simulink library "Actuator_AC_Lib"  (R2019b)
settings: Solver=VariableStepAuto  StartTime=0.0  StopTime=10.0  RelTol=1e-3
undefined symbols (not defined in the file): APN_Param
libraries: simulink x3, powerlib x2, electricdrivelib x1
Description:
  | Copyright 2019 The MathWorks, Inc.
settings Model: Creator=smiller  LastModifiedBy=smiller
settings SFSimCC: CustomCodeUndefinedFunction=UseInterfaceOnly

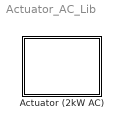
== system Actuator_AC_Lib ==
  Actuator (2kW AC) : Subsystem  VariantControlMode=Label  Variant=on  LabelModeActiveChoice=Phasor  mask{ModelType=Phasor, PQ_Model=Initial}
      mask prompts: ModelType "Model Type"; PQ_Model "PQ Model"
      mask init:
      | set_param(gcb,'LabelModeActiveChoice',get_param(gcb,'ModelType'));
      | set_param([gcb '/Phasor'],'PQ_Model',get_param(gcb,'PQ_Model'));
      settings: AttributesFormatString=%<BlockChoice>
      mask TypeOptions ModelType: Detailed | Phasor
      mask TypeOptions PQ_Model: Initial | Tuned
      mask Display:
      | blk=find_system(gcbh, 'SearchDepth', 1,'FollowLinks','on', 'LookUnderMasks','all', 'Parent', gcb,'VariantObject', get_param(gcb,'activevariant'));
      | eval(get_param(blk, 'MaskDisplay'));

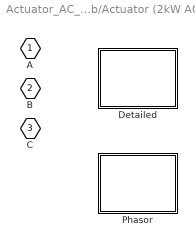
== system Actuator_AC_Lib/Actuator (2kW AC) ==
  Detailed : Subsystem  VariantControl=Detailed
      mask Display: image(imread('ActuatorAC_Detailed_IMAGE.jpg'));
  Phasor : Subsystem  VariantControl=Phasor  mask{PQ_Model=Initial}
      mask prompts: PQ_Model "PQ Model"
      mask init:
      | set_param([gcb '/Calc PQ'],'PQ_Model',get_param(gcb,'PQ_Model'));
      mask TypeOptions PQ_Model: Initial | Tuned
      mask Display: image('ActuatorAC_Phasor_IMAGE.jpg');
  A : PMIOPort  Side=Left
  B : PMIOPort  Port=2  Side=Left
  C : PMIOPort  Port=3  Side=Left

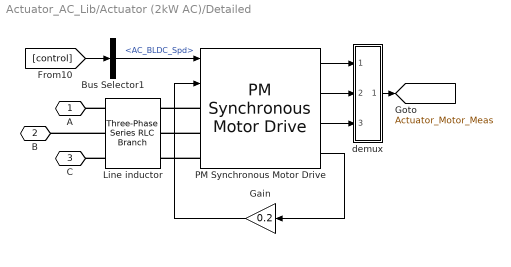
== system Actuator_AC_Lib/Actuator (2kW AC)/Detailed ==
  Bus Selector1 : BusSelector  OutputSignals=AC_BLDC_Spd
  Gain : Gain  Gain=0.2
  Line inductor : powerlib/Elements/Three-Phase Series RLC Branch  LConnTagsString=A|B|C  RConnTagsString=A|B|C  BranchType=L  Resistance=[]  Inductance=1e-3  Capacitance=[]  Measurements=None
      settings: SourceProductName=Simscape Electrical
  PM Synchronous Motor Drive : electricdrivelib/AC drives/PM Synchronous Motor Drive  Rs=0.2  Lls=8.5e-3  Lms=8.5e-3  MachineConstant=Flux linkage established by magnets (V.s)  FluxCst=0.175  VoltageCst=126.966  TorqueCst=1.05  ia=0  ib=0  J=0.089  Friction=0.005  p=4  wm=0  thetam=0  Rsnb_rec=10e3  Csnb_rec=20e-9  Ron_rec=1e-3  Vf_rec=1.3  cap_bus=2000e-6  Rbrake=8  fbrake=4000  activationVoltage=320  shutdownVoltage=310  sourceFrequency=60  deviceType=IGBT / Diodes  Ron_inv=1e-3  Vf_inv=0.8  Vfd_inv=0.8  Tf=1e-6  Tt=2e-6  Tf_GTO=0  Tt_GTO=0  Rsnb_inv=5000  Csnb_inv=inf  regulationType=Speed regulation  Acc=1000  Dec=-1000  kp_sc=5  ki_sc=100  fc_sc=100  Tsc=7*20e-6  Tmin=-17.8  Tmax=17.8  modulationType=Hysteresis  h=0.1  kp_Id=200  ki_Id=1000  kp_Iq=200  ki_Iq=1000  fc_bus=50  car_freq=20000  freq_max=20e3  Tvect=20e-6  zeta=0.9  Trd=0.1  bwRatio=30  baseSampleTime=2e-06  outputBusMode=Multiple output buses  busLabels=off  MechanicalLoad=Torque Tm  modelDetailLevel=Detailed  driveType=AC6  AverageValue=off
      settings: SourceProductName=Simscape Electrical  SourceProductBaseCode=PS
  demux : Subsystem
  A : PMIOPort  Side=Left
  B : PMIOPort  Port=2  Side=Left
  C : PMIOPort  Port=3  Side=Left
  tag scope: Actuator_Motor_Meas=global
  wires:
  PM Synchronous Motor Drive/3 -> demux/3(Ctrl)
  PM Synchronous Motor Drive/2 -> demux/2(Conv.)
  PM Synchronous Motor Drive/1 -> demux/1(motor)
  PM Synchronous Motor Drive/4 -> Gain/1
  Gain/1 -> PM Synchronous Motor Drive/2
  Bus Selector1/1 -> PM Synchronous Motor Drive/1  "<AC_BLDC_Spd>"
  demux/1(S) -> [Actuator_Motor_Meas]
  [control] -> Bus Selector1/1
  connections:
  Line inductor/LConn1 -- A/RConn1
  Line inductor/LConn2 -- B/RConn1
  Line inductor/LConn3 -- C/RConn1
  PM Synchronous Motor Drive/LConn1 -- Line inductor/RConn1
  PM Synchronous Motor Drive/LConn2 -- Line inductor/RConn2
  PM Synchronous Motor Drive/LConn3 -- Line inductor/RConn3

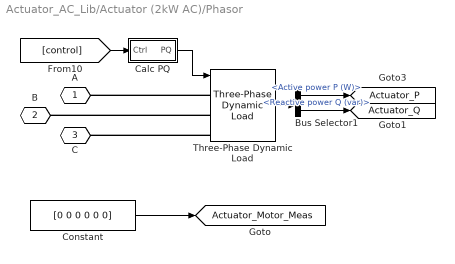
== system Actuator_AC_Lib/Actuator (2kW AC)/Phasor ==
  Bus Selector1 : BusSelector  OutputSignals=Active power P (W),Reactive power Q (var)
  Calc PQ : Subsystem  VariantControlMode=Label  Variant=on  LabelModeActiveChoice=Initial  mask{PQ_Model=Initial}
      mask prompts: PQ_Model "PQ Model"
      mask init:
      | set_param(gcb,'LabelModeActiveChoice',get_param(gcb,'PQ_Model'));
      settings: AttributesFormatString=%<LabelModeActiveChoice>
      mask TypeOptions PQ_Model: Initial | Tuned
      mask Display: disp(' ');
  Constant : Constant  Value=[0 0 0 0 0 0]
  Three-Phase Dynamic Load : powerlib/Elements/Three-Phase Dynamic Load  NominalVoltage=[ 500e3 400 ]  ActiveReactivePowers=[APN_Param.Actuator.P APN_Param.Actuator.Q]  PositiveSequence=[0.0004 0]  ExternalControl=on  NpNq=[1.3 2]  TimeConstants="[0  0  0  0]"  MinimumVoltage=0.7  Tfilter=1e-4  LoadFlowParameters=[4,0,0,0,0]
      settings: SourceProductName=Simscape Electrical  SourceProductBaseCode=PS
  A : PMIOPort  Side=Left
  B : PMIOPort  Port=2  Side=Left
  C : PMIOPort  Port=3  Side=Left
  tag scope: Actuator_Motor_Meas=global, Actuator_P=global, Actuator_Q=global
  wires:
  Bus Selector1/1 -> [Actuator_P]  "<Active power P (W)>"
  Three-Phase Dynamic Load/1 -> Bus Selector1/1
  Calc PQ/1(PQ) -> Three-Phase Dynamic Load/1
  Constant/1 -> [Actuator_Motor_Meas]
  Bus Selector1/2 -> [Actuator_Q]  "<Reactive power Q (var)>"
  [control] -> Calc PQ/1(Ctrl)
  connections:
  Three-Phase Dynamic Load/LConn3 -- C/RConn1
  Three-Phase Dynamic Load/LConn1 -- A/RConn1
  Three-Phase Dynamic Load/LConn2 -- B/RConn1

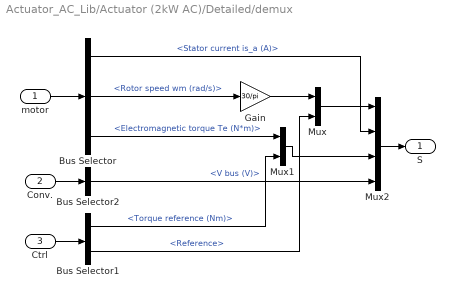
== system Actuator_AC_Lib/Actuator (2kW AC)/Detailed/demux ==
  motor : Inport
  Conv. : Inport  Port=2
  Ctrl : Inport  Port=3
  Bus Selector : BusSelector  OutputSignals=Stator current is_a (A),Rotor speed wm (rad/s),Electromagnetic torque Te (N*m)
  Bus Selector1 : BusSelector  OutputSignals=Torque reference (Nm),Reference
  Bus Selector2 : BusSelector  OutputSignals=V bus (V)
  Gain : Gain  Gain=30/pi  SaturateOnIntegerOverflow=on  OutDataTypeStr=Inherit: Same as input  ParamDataTypeStr=Inherit: Same as input
  Mux : Mux  Inputs=2
  Mux1 : Mux  Inputs=2
  Mux2 : Mux
  S : Outport  VectorParamsAs1DForOutWhenUnconnected=off
  wires:
  motor/1 -> Bus Selector/1
  Mux/1 -> Mux2/2
  Mux1/1 -> Mux2/3
  Bus Selector/3 -> Mux1/1  "<Electromagnetic torque Te (N*m)>"
  Bus Selector/1 -> Mux2/1  "<Stator current is_a (A)>"
  Gain/1 -> Mux/1
  Bus Selector1/2 -> Mux/2  "<Reference>"
  Bus Selector1/1 -> Mux1/2  "<Torque reference (Nm)>"
  Ctrl/1 -> Bus Selector1/1
  Conv./1 -> Bus Selector2/1
  Bus Selector2/1 -> Mux2/4  "<V bus (V)>"
  Bus Selector/2 -> Gain/1  "<Rotor speed wm (rad/s)>"
  Mux2/1 -> S/1

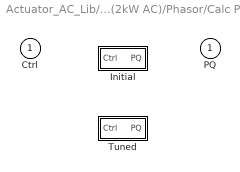
== system Actuator_AC_Lib/Actuator (2kW AC)/Phasor/Calc PQ ==
  Ctrl : Inport
  Initial : Subsystem  VariantControl=Initial
  Tuned : Subsystem  VariantControl=Tuned
  PQ : Outport  VectorParamsAs1DForOutWhenUnconnected=off

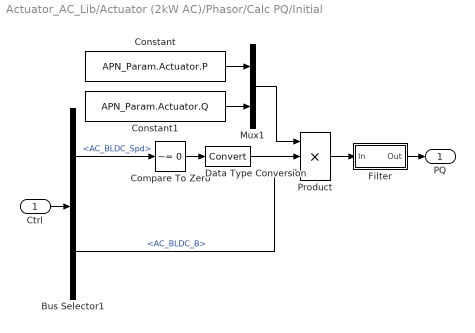
== system Actuator_AC_Lib/Actuator (2kW AC)/Phasor/Calc PQ/Initial ==
  Ctrl : Inport
  Bus Selector1 : BusSelector  OutputSignals=AC_BLDC_Spd,AC_BLDC_B
  Compare To Zero : simulink/Logic and Bit Operations/Compare To Zero  relop=~=  OutDataTypeStr=boolean
  Constant : Constant  Value=APN_Param.Actuator.P
  Constant1 : Constant  Value=APN_Param.Actuator.Q
  Data Type Conversion : DataTypeConversion
  Filter : Subsystem  mask(First-order lag supporting vector signals){b=1e-2, x_initial=[APN_Param.Actuator.P APN_Param.Actuator.Q]*0}
      mask prompts: b "Filter time constant"; x_initial "Initial output"
      mask help: Models a lag of the form 1/(b*s+1) where s is the Laplace operator.
  Mux1 : Mux  Inputs=2
  Product : Product  Inputs=3
  PQ : Outport  VectorParamsAs1DForOutWhenUnconnected=off
  wires:
  Filter/1(Out) -> PQ/1
  Bus Selector1/2 -> Product/3  "<AC_BLDC_B>"
  Bus Selector1/1 -> Compare To Zero/1  "<AC_BLDC_Spd>"
  Ctrl/1 -> Bus Selector1/1
  Compare To Zero/1 -> Data Type Conversion/1
  Data Type Conversion/1 -> Product/2
  Mux1/1 -> Product/1
  Constant/1 -> Mux1/1
  Constant1/1 -> Mux1/2
  Product/1 -> Filter/1(In)

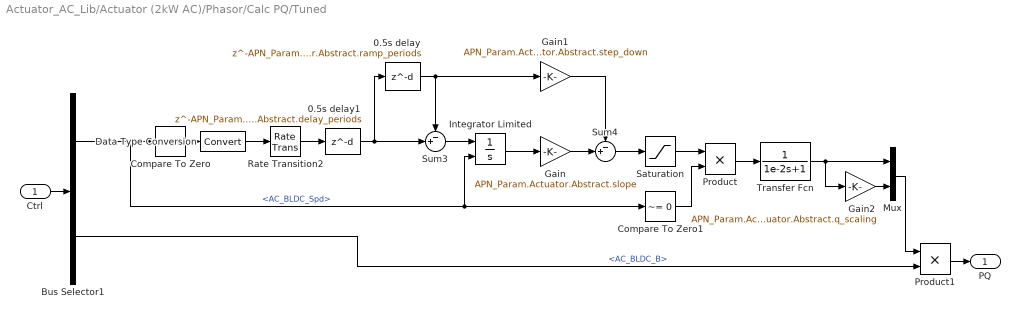
== system Actuator_AC_Lib/Actuator (2kW AC)/Phasor/Calc PQ/Tuned ==
  Ctrl : Inport
  0.5s delay : Delay  DelayLength=APN_Param.Actuator.Abstract.ramp_periods  SampleTime=0.01
  0.5s delay1 : Delay  DelayLength=APN_Param.Actuator.Abstract.delay_periods  SampleTime=0.01
  Bus Selector1 : BusSelector  OutputSignals=AC_BLDC_Spd,AC_BLDC_B
  Compare To Zero : simulink/Logic and Bit Operations/Compare To Zero  relop=~=  OutDataTypeStr=boolean
  Compare To Zero1 : simulink/Logic and Bit Operations/Compare To Zero  relop=~=  OutDataTypeStr=boolean
  Data Type Conversion : DataTypeConversion
  Gain : Gain  Gain=APN_Param.Actuator.Abstract.slope
  Gain1 : Gain  Gain=APN_Param.Actuator.Abstract.step_down
  Gain2 : Gain  Gain=APN_Param.Actuator.Abstract.q_scaling
  Integrator Limited : Integrator  ExternalReset=falling  LimitOutput=on  UpperSaturationLimit=1  LowerSaturationLimit=0
  Mux : Mux  Inputs=2
  Product : Product
  Product1 : Product
  Rate Transition2 : RateTransition  OutPortSampleTime=0.01
  Saturation : Saturate  UpperLimit=1160  LowerLimit=0
  Sum3 : Sum  Inputs=-+|  SaturateOnIntegerOverflow=on  InputSameDT=on  OutDataTypeStr=Inherit: Same as first input
  Sum4 : Sum  Inputs=-+|  SaturateOnIntegerOverflow=on  InputSameDT=on  OutDataTypeStr=Inherit: Same as first input
  Transfer Fcn : TransferFcn  Denominator=[1e-2 1]
  PQ : Outport  VectorParamsAs1DForOutWhenUnconnected=off
  wires:
  Compare To Zero1/1 -> Product/2
  Saturation/1 -> Product/1
  Sum4/1 -> Saturation/1
  0.5s delay/1 -> Gain1/1, Sum3/1
  Gain1/1 -> Sum4/1
  Product/1 -> Transfer Fcn/1
  Sum3/1 -> Integrator Limited/1
  Rate Transition2/1 -> 0.5s delay1/1
  Gain/1 -> Sum4/2
  Data Type Conversion/1 -> Rate Transition2/1
  Integrator Limited/1 -> Gain/1
  Compare To Zero/1 -> Data Type Conversion/1
  Transfer Fcn/1 -> Gain2/1, Mux/1
  Ctrl/1 -> Bus Selector1/1
  Gain2/1 -> Mux/2
  Mux/1 -> Product1/1
  Bus Selector1/1 -> Integrator Limited/2, Compare To Zero1/1, Compare To Zero/1  "<AC_BLDC_Spd>"
  0.5s delay1/1 -> Sum3/2, 0.5s delay/1
  Bus Selector1/2 -> Product1/2  "<AC_BLDC_B>"
  Product1/1 -> PQ/1

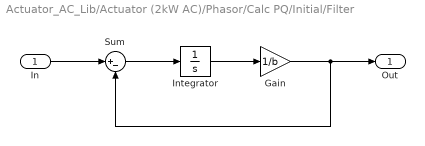
== system Actuator_AC_Lib/Actuator (2kW AC)/Phasor/Calc PQ/Initial/Filter ==
  In : Inport
  Gain : Gain  Gain=1/b
  Integrator : Integrator  InitialCondition=x_initial
  Sum : Sum  Inputs=|+-  SaturateOnIntegerOverflow=on  InputSameDT=on  OutDataTypeStr=Inherit: Same as first input
  Out : Outport  VectorParamsAs1DForOutWhenUnconnected=off
  wires:
  Gain/1 -> Out/1, Sum/2
  Integrator/1 -> Gain/1
  In/1 -> Sum/1
  Sum/1 -> Integrator/1
